simulink model "magnetic_field_loop"  (R2026a)
settings: Solver=VariableStepAuto  StopTime=5200
undefined symbols (not defined in the file): IAU, juliandate, WMM2025
libraries: aerolibtransform2 x3, simulink x2, matrix_library x1, simulink_extras x1, aerolibgravity2 x1, dspfdesign x1, aerolibutil x1
settings Model: SimulationMode=accelerator  Creator=2728308h  LastModifiedBy=2728308h

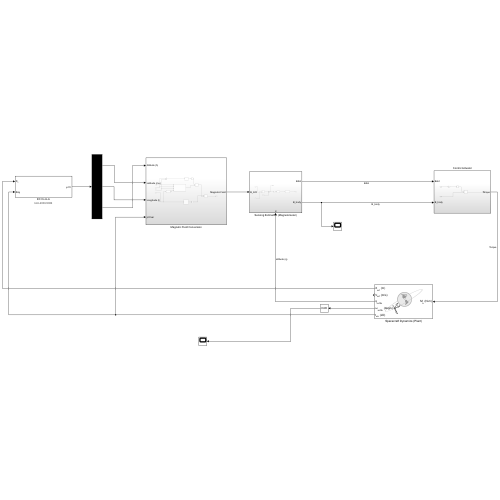
[thumbnail: Simulink's stored preview of the top-level diagram]
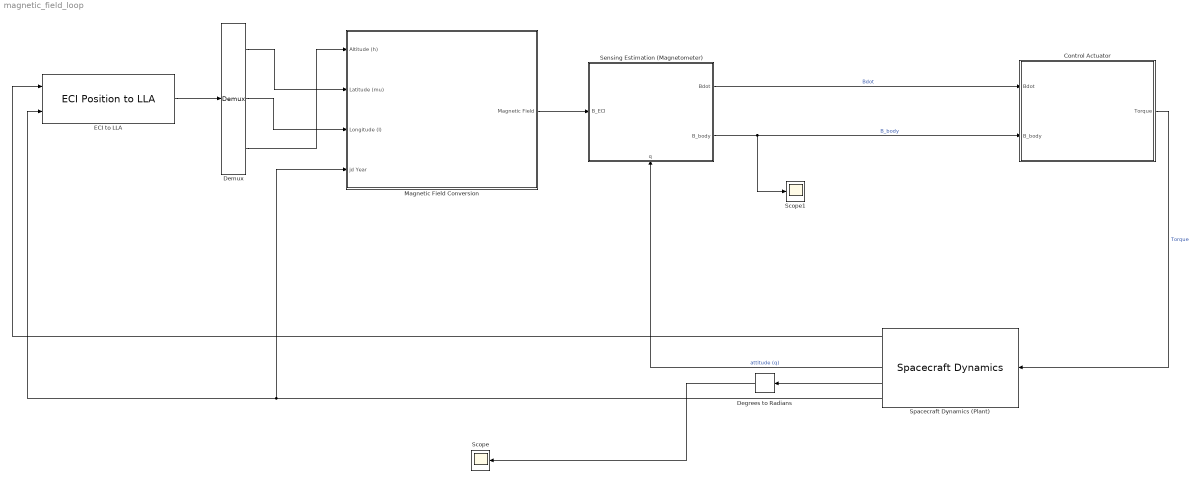
== system magnetic_field_loop ==
  Control Actuator : Subsystem
  Degrees to Radians : simulink_extras/Transformations/Degrees to Radians
  Demux : Demux  Outputs=3
  ECI to LLA : aerolibtransform2/ECI Position to LLA  red=IAU-2000/2006  year=2013  month=January  day=1  hour=0  min=0  sec=0  deltaT=Day  errorflag=Error  extraparamflag=off  eunits=Metric (MKS)  earthmodel=WGS84  flat=1/298.257223563  eqradius=6378137
      settings: AttributesFormatString=%<red>
  Magnetic Field Conversion : Subsystem
  Scope : Scope
      settings: ActiveDisplayYMinimum=-423935.52919452224  ActiveDisplayYMaximum=593401.71213267965
  Scope1 : Scope
  Sensing Estimation (Magnetometer) : Subsystem
      settings: PortSchema="{\"entries\":[{\"content\":{\"sides\":[{\"content\":{\"connectorIds\":[\"In1\"]},\"type\":\"ConnectorPlacement.EquallySpacedRectSide\",\"uuid\":\"50d83977-9467-45f1-a90f-e49ea50c9f9d\"},{\"content\":{\"connectorIds\":[\"Out1\",\"Out2\"],\"side\":\"RIGHT\"},\"type\":\"ConnectorPlacement.EquallySpacedRectSide\",\"uuid\":\"0f78f750-bdbd-4412-b85f-71581e999bb5\"},{\"content\":{\"side\":\"TOP\"},\"type\":\"ConnectorPlacement.EquallySpacedRectSide\",\"uuid\":\"888d3c08-f478-40dd-b4d8-06463caf1981\"},{\"content\":{\"connectorIds\":[\"In2\"],\"side\":\"BOTTOM\"},\"type\":\"ConnectorPlacement.EquallySpacedRectSide\",\"uuid\":\"cd8cedf7-0646-4c45-ac4e-e3720e525f1f\"}]},\"type\":\"ConnectorPlacement.EquallySpacedConnector\",\"uuid\":\"9105679a-e235-40a2-a213-9c6ee0154039\"}],\"packageUris\":[\"http://schema.mathworks.com/mf0/Connector/R2020b\"],\"version\":\"1.0\"}"
  Spacecraft Dynamics (Plant) : SpacecraftDynamics  forcesIn=off  startDate=juliandate(2025, 1, 1, 12, 0, 0)  attitudeRate=[2, 3, 4]
  wires:
  Spacecraft Dynamics (Plant)/3 -> Sensing Estimation (Magnetometer)/2(q)  "attitude (q)"
  Sensing Estimation (Magnetometer)/1(Bdot) -> Control Actuator/1(Bdot)  "Bdot"
  Control Actuator/1(Torque) -> Spacecraft Dynamics (Plant)/1  "Torque"
  Magnetic Field Conversion/1(Magnetic Field) -> Sensing Estimation (Magnetometer)/1(B_ECI)
  ECI to LLA/1 -> Demux/1
  Demux/1 -> Magnetic Field Conversion/2(Latitude (mu))
  Demux/2 -> Magnetic Field Conversion/3(Longitude (I))
  Demux/3 -> Magnetic Field Conversion/1(Altitude (h))
  Spacecraft Dynamics (Plant)/5 -> Magnetic Field Conversion/4(jd Year), ECI to LLA/2
  Spacecraft Dynamics (Plant)/1 -> ECI to LLA/1
  Sensing Estimation (Magnetometer)/2(B_body) -> Scope1/1, Control Actuator/2(B_body)  "B_body"
  Degrees to Radians/1 -> Scope/1
  Spacecraft Dynamics (Plant)/4 -> Degrees to Radians/1

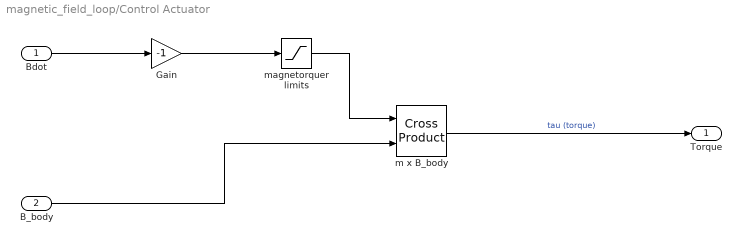
== system magnetic_field_loop/Control Actuator ==
  Bdot : Inport
  B_body : Inport  Port=2
  Gain : Gain  Gain=-1
  m x B_body : matrix_library/Cross Product
  magnetorquer limits : Saturate
  Torque : Outport
  wires:
  Bdot/1 -> Gain/1
  Gain/1 -> magnetorquer limits/1
  magnetorquer limits/1 -> m x B_body/1
  B_body/1 -> m x B_body/2
  m x B_body/1 -> Torque/1  "tau (torque)"

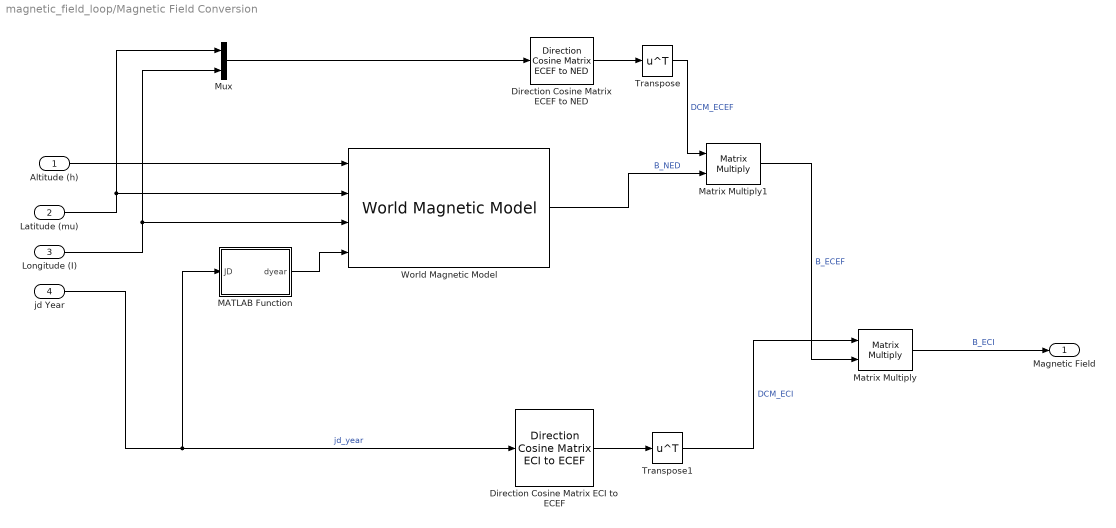
== system magnetic_field_loop/Magnetic Field Conversion ==
  Altitude (h) : Inport
  Latitude (mu) : Inport  Port=2
  Longitude (I) : Inport  Port=3
  jd Year : Inport  Port=4
  Direction Cosine Matrix ECEF to NED : aerolibtransform2/Direction Cosine Matrix ECEF to NED
  Direction Cosine Matrix ECI to ECEF : aerolibtransform2/Direction Cosine Matrix ECI to ECEF  red=IAU-2000/2006  year=2013  month=January  day=1  hour=0  min=0  sec=0  deltaT=Day  errorflag=Error  extraparamflag=off
      settings: AttributesFormatString=%<red>
  MATLAB Function : MATLAB Function  TreatAsAtomicUnit=on
  Matrix Multiply : Product  Multiplication=Matrix(*)
  Matrix Multiply1 : Product  Multiplication=Matrix(*)
  Mux : Mux  Inputs=2
  Transpose : Math  Operator=transpose
  Transpose1 : Math  Operator=transpose
  World Magnetic Model : aerolibgravity2/World Magnetic Model  model=WMM2025 (2025-2030)  customFile='WMM2025.COF'  units=Metric (MKS)  time_in=on  month=January  day=1  year=2025  action=Error  h_out=off  dec_out=off  inc_out=off  ti_out=off
  Magnetic Field : Outport
  wires:
  Altitude (h)/1 -> World Magnetic Model/1
  jd Year/1 -> MATLAB Function/1(JD), Direction Cosine Matrix ECI to ECEF/1  "jd_year"
  Longitude (I)/1 -> World Magnetic Model/3, Mux/2
  Direction Cosine Matrix ECEF to NED/1 -> Transpose/1
  Direction Cosine Matrix ECI to ECEF/1 -> Transpose1/1
  Transpose1/1 -> Matrix Multiply/1  "DCM_ECI"
  Matrix Multiply/1 -> Magnetic Field/1  "B_ECI"
  Latitude (mu)/1 -> World Magnetic Model/2, Mux/1
  Mux/1 -> Direction Cosine Matrix ECEF to NED/1
  World Magnetic Model/1 -> Matrix Multiply1/2  "B_NED"
  Transpose/1 -> Matrix Multiply1/1  "DCM_ECEF"
  Matrix Multiply1/1 -> Matrix Multiply/2  "B_ECEF"
  MATLAB Function/1(dyear) -> World Magnetic Model/4

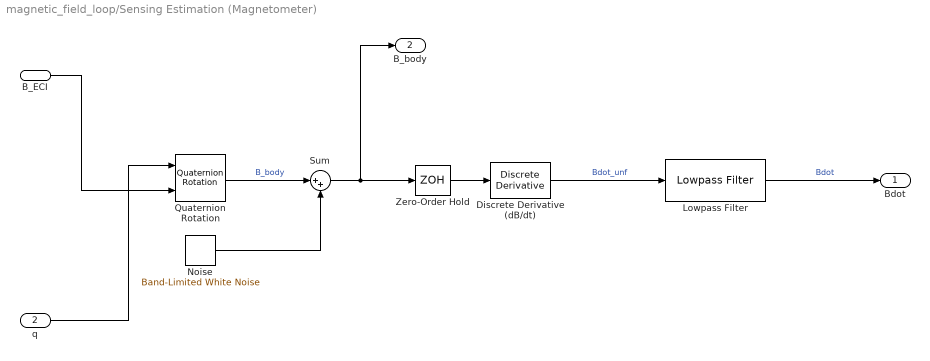
== system magnetic_field_loop/Sensing Estimation (Magnetometer) ==
  B_ECI : Inport
  q : Inport  Port=2
  Discrete Derivative (dB/dt) : simulink/Discrete/Discrete Derivative  gainval=1.0  ICPrevScaledInput=0.0  OutMin=[]  OutMax=[]  OutDataType=fixdt(1, 16)  OutScaling=2^-10  DoSatur=off
  Lowpass Filter : dspfdesign/Lowpass Filter  FilterType=FIR  DesignForMinimumOrder=on  FilterOrder=50  PassbandFrequency=0.3628  StopbandFrequency=0.5442  PassbandRipple=0.1  StopbandAttenuation=80  SampleRateMode=Use normalized frequency (0 to 1)  SampleRate=44100  SimulateUsing=Interpreted execution  roundingMode=Floor  coeffsDataTypeStr=fixdt(1,16)
  Noise : simulink/Sources/Band-Limited White Noise  Cov=[0.1]  Ts=0.1  seed=[23341]
  Quaternion Rotation : aerolibutil/Quaternion Rotation
  Sum : Sum  Inputs=|++
  Zero-Order Hold : ZeroOrderHold  SampleTime=-1
  Bdot : Outport
  B_body : Outport  Port=2
  wires:
  q/1 -> Quaternion Rotation/1
  B_ECI/1 -> Quaternion Rotation/2
  Quaternion Rotation/1 -> Sum/1  "B_body"
  Noise/1 -> Sum/2
  Sum/1 -> Zero-Order Hold/1, B_body/1
  Lowpass Filter/1 -> Bdot/1  "Bdot"
  Discrete Derivative (dB/dt)/1 -> Lowpass Filter/1  "Bdot_unf"
  Zero-Order Hold/1 -> Discrete Derivative (dB/dt)/1

== matlab function magnetic_field_loop/Magnetic Field Conversion/MATLAB Function ==
  data: JD input; dyear output
function dyear = jd2decyear(JD)
%julian date of Jan 1, 2000, 00:00 UTC (reference)in dec
JD2000 = 2451544.5;

%days since that reference
daysSince2000 = JD - JD2000;

%approximate year
yr = 2000 + floor(daysSince2000 / 365.25);

%julian date at Jan 1, 00:00 UTC of that approximate year
JDstartOfYear = JD2000 + 365*(yr-2000) + floor((yr-2000)/4) - floor((yr-2000)/100) + floor((yr-2000)/400);

%correct year
while JD < JDstartOfYear
    yr = yr - 1;
    JDstartOfYear = JD2000 + 365*(yr-2000) + floor((yr-2000)/4) - floor((yr-2000)/100) + floor((yr-2000)/400);
end
isLeap = (mod(yr,4)==0 && mod(yr,100)~=0) || mod(yr,400)==0;
daysInYear = 365 + double(isLeap);

dyear = yr + (JD - JDstartOfYear) / daysInYear;
end
